simulink model "CTDSM_CIFF_SECOND_2048_RESIDUAL_OFFSET_CHOPPING"  (R2025b)
settings: Solver=VariableStepAuto  StartTime=0.0  StopTime=0.5  RelTol=1e-3
libraries: fl_lib x13, nesl_utility x6, ee_lib x2, simulink_extras x1, cstblocks x1, dspobslib x1
settings Model: Creator=Team_33  LastModifiedBy=k2vas

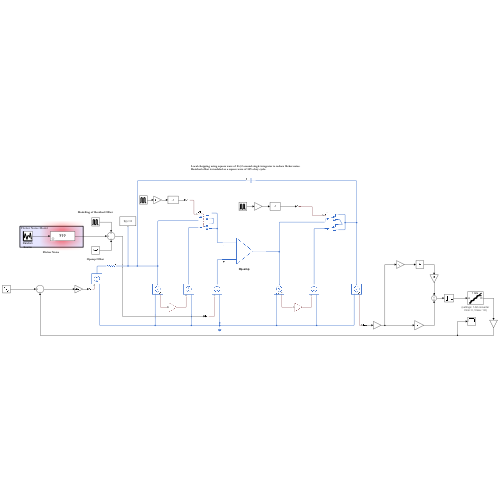
[thumbnail: Simulink's stored preview of the top-level diagram]
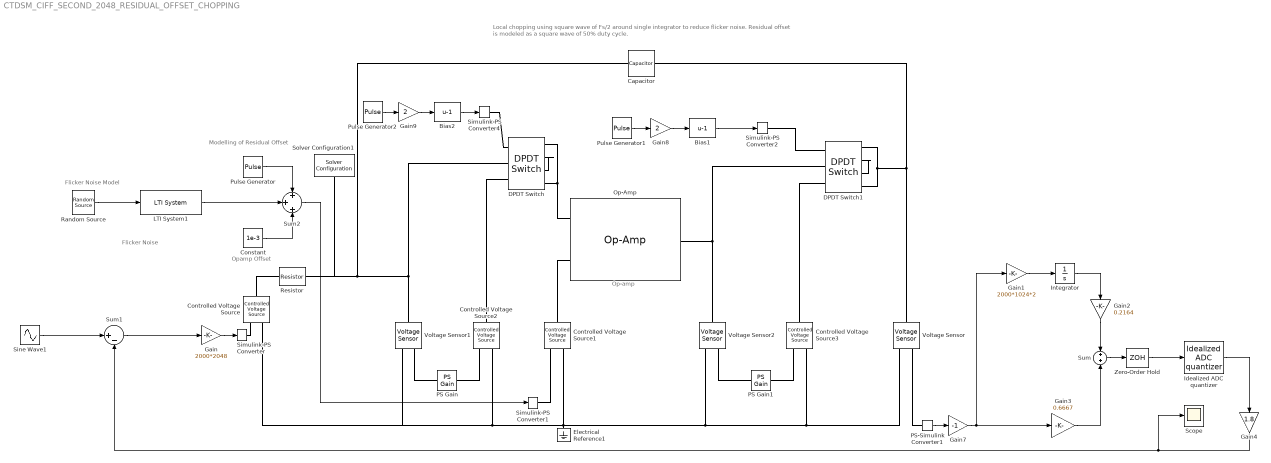
== system CTDSM_CIFF_SECOND_2048_RESIDUAL_OFFSET_CHOPPING ==
  note: Op-amp
  note: Local chopping using square wave of Fs/2 around single integrator to reduce flicker noise. Residual offset is modeled as a square wave of 50% duty cycle.
  note: Flicker Noise Model
  note: Opamp Offset
  note: Flicker Noise
  note: Modelling of Residual Offset
  Bias1 : Bias  Bias=-1  SaturateOnIntegerOverflow=off
  Bias2 : Bias  Bias=-1  SaturateOnIntegerOverflow=off
  Capacitor : fl_lib/Electrical/Electrical Elements/Capacitor  c=1 F  r=0 Ohm  g=0 1/Ohm  i_specify=off  i_priority=None  i=0 A  i_nominal_specify=off  i_nominal_value=1  i_nominal_unit=A  v_specify=off  v_priority=None  v=0 V  v_nominal_specify=off  v_nominal_value=1  v_nominal_unit=V  vc_specify=off  vc_priority=High  vc=0 V  vc_nominal_specify=off  vc_nominal_value=1  vc_nominal_unit=V
  Constant : Constant  Value=1e-3
  Controlled Voltage Source{,1..3} (4 alike) : fl_lib/Electrical/Electrical Sources/Controlled Voltage Source
  DPDT Switch : ee_lib/Switches & Breakers/DPDT Switch  R_closed=0.01 Ohm  G_open=1e-6 S  Threshold=0.5 V  Width=0 V  model_dynamics=0  t_on=1e-3 s  t_off=1e-3 s  initial_vT=0 V
      settings: InternalSimscapePortConfiguration="{\"Bottom\":[],\"Left\":[{\"id\":\"vT\",\"label\":\"vT\",\"type\":\"input\"},{\"id\":\"p1\",\"label\":\"\",\"type\":\"foundation.electrical.electrical\"},{\"id\":\"p2\",\"label\":\"\",\"type\":\"foundation.electrical.electrical\"}],\"Right\":[{\"id\":\"n11\",\"label\":\"\",\"type\":\"foundation.electrical.electrical\"},{\"id\":\"n12\",\"label\":\"\",\"type\":\"foundation.electrical.electrical\"},{\"id\":\"n21\",\"label\":\"\",\"type\":\"foundation.electrical.electrical\"},{\"id\":\"n22\",\"label\":\"\",\"type\":\"foundation.electrical.electrical\"}],\"Top\":[]}"
  DPDT Switch1 : ee_lib/Switches & Breakers/DPDT Switch  R_closed=0.01 Ohm  G_open=1e-6 S  Threshold=0.5 V  Width=0 V  model_dynamics=0  t_on=1e-3 s  t_off=1e-3 s  initial_vT=0 V
      settings: InternalSimscapePortConfiguration="{\"Bottom\":[],\"Left\":[{\"id\":\"vT\",\"label\":\"vT\",\"type\":\"input\"},{\"id\":\"p1\",\"label\":\"\",\"type\":\"foundation.electrical.electrical\"},{\"id\":\"p2\",\"label\":\"\",\"type\":\"foundation.electrical.electrical\"}],\"Right\":[{\"id\":\"n11\",\"label\":\"\",\"type\":\"foundation.electrical.electrical\"},{\"id\":\"n12\",\"label\":\"\",\"type\":\"foundation.electrical.electrical\"},{\"id\":\"n21\",\"label\":\"\",\"type\":\"foundation.electrical.electrical\"},{\"id\":\"n22\",\"label\":\"\",\"type\":\"foundation.electrical.electrical\"}],\"Top\":[]}"
  Electrical Reference1 : fl_lib/Electrical/Electrical Elements/Electrical Reference
  Gain : Gain  Gain=2000*2048
  Gain1 : Gain  Gain=2000*1024*2
  Gain2 : Gain  Gain=0.2164
  Gain3 : Gain  Gain=0.6667
  Gain4 : Gain  Gain=1.8
  Gain7 : Gain  Gain=-1
  Gain8 : Gain  Gain=2
  Gain9 : Gain  Gain=2
  Idealized ADC quantizer : simulink_extras/Additional Discrete/Idealized ADC quantizer  NumberOfConverterBits=1  Vmin=0  Vmax=1.8  OutputDataType=int16  OutputNegativeValues=off
  Integrator : Integrator
  LTI System1 : cstblocks/LTI System  sys=ff_ss  IC=[]  PadeOrder=0
  Op-Amp : fl_lib/Electrical/Electrical Elements/Op-Amp  outI_specify=off  outI_priority=None  outI=0 A  outI_nominal_specify=off  outI_nominal_value=1  outI_nominal_unit=A
  PS Gain : fl_lib/Physical Signals/Functions/PS Gain  gain=-1
  PS Gain1 : fl_lib/Physical Signals/Functions/PS Gain  gain=-1
  PS-Simulink Converter1 : nesl_utility/PS-Simulink Converter  PhysicalDomain=network_engine_domain  SubClassName=ps_output  LeftPortType=input  RightPortType=output  PseudoPeriodic=off  Frequencies=[]  VectorFormat=inherit  Unit=inherit  AffineConversion=off
  Pulse Generator : DiscretePulseGenerator  PulseType=Time based  Amplitude=2  Period=2/(2000*2048)  PulseWidth=50
  Pulse Generator1 : DiscretePulseGenerator  PulseType=Time based  Period=2/(2000*2048)  PulseWidth=50
  Pulse Generator2 : DiscretePulseGenerator  PulseType=Time based  Period=2/(2048*2000)  PulseWidth=50
  Random Source : dspobslib/Random Source  SrcType=Gaussian  NormMethod=Ziggurat  CltLength=12  MinVal=0  MaxVal=1  MeanVal=0  VarVal=1e-8  RepMode=Not repeatable  rawSeed=1  IsInherit=off  SampMode=Continuous  SampTime=1/(2000*2048)  SampFrame=1  DataType=Double  OutComplex=Real  OutputFrames=off
  Resistor : fl_lib/Electrical/Electrical Elements/Resistor  R=1 Ohm  i_specify=off  i_priority=None  i=0 A  i_nominal_specify=off  i_nominal_value=1  i_nominal_unit=A  v_specify=off  v_priority=None  v=0 V  v_nominal_specify=off  v_nominal_value=1  v_nominal_unit=V
  Scope : Scope
      settings: ActiveDisplayYMinimum=-0.225  ActiveDisplayYMaximum=2.02499  DataLoggingVariableName=output_data  DataLoggingSaveFormat=Array
  Simulink-PS Converter{,1..2,4} (4 alike) : nesl_utility/Simulink-PS Converter  PhysicalDomain=network_engine_domain  SubClassName=ps_input  LeftPortType=input  RightPortType=output  PseudoPeriodic=off  Frequencies=[]  NoiseDistribution=none  NoiseParameters=[]  Unit=1  AffineConversion=off  FilteringAndDerivatives=provide  SimscapeFilterOrder=1  InputFilterTimeConstant=0.001  UdotUserProvided=0
  Sine Wave1 : Sin  Amplitude=0.5  Bias=0.9  Frequency=((2000*1024)*127*2*2*pi)/(32768*32)  SampleTime=0
  Solver Configuration1 : nesl_utility/Solver Configuration  PhysicalDomain=network_engine_domain  SubClassName=solver  LeftPortType=input  RightPortType=generic  Tones=[]  Harmonics=[]  SimulateNoise=off  Profile=off  UseLocalSampling=off  EnableSwitchedLinearOptims=on  FrequencyDomain=off  UseCCode=off  RelTol=0.001  AbsTol=0.001  MinStep=1e-09  ToWorkspace=off  RevertToSquareIcSolve=off  NumHomotopyIterations=100  PhasorMode=off  PhasorModeNumHarmonics=1  ConsistencySolver=NEWTON_XTOL_AFTER_FTOL  IndexReductionMethod=DerivativeReplacement  DoDC=off  ResidualTolerance=1e-09  ConsistencyTolSource=GLOBAL  ConsistencyAbsTol=0.001  ConsistencyRelTol=0.001  ConsistencyTolFactor=0.001  UseLocalSolver=off  LocalSolverChoice=NE_BACKWARD_EULER_ADVANCER  ResolveIndetEquations=on  FunctionEvalNumThread=1  LocalSolverSampleTime=0.001  DoFixedCost=off  MaxNonlinIter=3  MaxModeIter=2  ComputeImpulses=off  ImpulseIterations=2  LinearAlgebra=auto  LinearAlgebraNumThread=0  EquationFormulation=NE_TIME_EF  DelaysMemoryBudget=1024  AutomaticFiltering=on  FilteringTimeConstant=0.001  PartitionStorageMethod=AS_NEEDED  PartitionMemoryBudget=1024  PartitionMethod=ROBUST  MultibodyUseLocalSolver=off  MultibodyLocalSolverChoice=ODE1  MultibodyLocalSolverSampleTime=0.001
  Sum : Sum  Inputs=+|+
  Sum1 : Sum  Inputs=|+-
  Sum2 : Sum  Inputs=+|+|+
  Voltage Sensor : fl_lib/Electrical/Electrical Sensors/Voltage Sensor
  Voltage Sensor1 : fl_lib/Electrical/Electrical Sensors/Voltage Sensor
  Voltage Sensor2 : fl_lib/Electrical/Electrical Sensors/Voltage Sensor
  Zero-Order Hold : ZeroOrderHold  SampleTime=1/(2000*1024*2)
  wires:
  Sum1/1 -> Gain/1
  Gain2/1 -> Sum/1
  Gain3/1 -> Sum/2
  Gain/1 -> Simulink-PS Converter/1
  PS-Simulink Converter1/1 -> Gain7/1
  Zero-Order Hold/1 -> Idealized ADC quantizer/1
  Idealized ADC quantizer/1 -> Gain4/1
  Gain1/1 -> Integrator/1
  Gain4/1 -> Scope/1, Sum1/2
  Integrator/1 -> Gain2/1
  Sum/1 -> Zero-Order Hold/1
  Sine Wave1/1 -> Sum1/1
  Gain7/1 -> Gain1/1, Gain3/1
  Bias1/1 -> Simulink-PS Converter2/1
  Pulse Generator1/1 -> Gain8/1
  Gain8/1 -> Bias1/1
  Pulse Generator2/1 -> Gain9/1
  Bias2/1 -> Simulink-PS Converter4/1
  Gain9/1 -> Bias2/1
  Random Source/1 -> LTI System1/1
  LTI System1/1 -> Sum2/2
  Pulse Generator/1 -> Sum2/1
  Sum2/1 -> Simulink-PS Converter1/1
  Constant/1 -> Sum2/3
  connections:
  DPDT Switch1/RConn1 -- DPDT Switch1/RConn4 -- Capacitor/RConn1 -- Voltage Sensor/LConn1
  Controlled Voltage Source/LConn1 -- Resistor/LConn1
  PS-Simulink Converter1/LConn1 -- Voltage Sensor/RConn1
  Controlled Voltage Source/RConn1 -- Simulink-PS Converter/RConn1
  Voltage Sensor/RConn2 -- Controlled Voltage Source3/RConn2 -- Voltage Sensor2/RConn2 -- Electrical Reference1/LConn1 -- Controlled Voltage Source1/RConn2 -- Voltage Sensor1/RConn2 -- Controlled Voltage Source/RConn2 -- Controlled Voltage Source2/RConn2
  DPDT Switch/RConn1 -- Op-Amp/LConn2 -- DPDT Switch/RConn4
  DPDT Switch/RConn2 -- DPDT Switch/RConn3
  Simulink-PS Converter4/RConn1 -- DPDT Switch/LConn1
  DPDT Switch1/LConn1 -- Simulink-PS Converter2/RConn1
  Voltage Sensor1/RConn1 -- PS Gain/LConn1
  PS Gain/RConn1 -- Controlled Voltage Source2/RConn1
  Voltage Sensor2/RConn1 -- PS Gain1/LConn1
  PS Gain1/RConn1 -- Controlled Voltage Source3/RConn1
  DPDT Switch1/RConn2 -- DPDT Switch1/RConn3
  Controlled Voltage Source1/LConn1 -- Op-Amp/LConn1
  Controlled Voltage Source1/RConn1 -- Simulink-PS Converter1/RConn1
  Voltage Sensor1/LConn1 -- DPDT Switch/LConn2 -- Capacitor/LConn1 -- Solver Configuration1/RConn1 -- Resistor/RConn1
  Controlled Voltage Source2/LConn1 -- DPDT Switch/LConn3
  Controlled Voltage Source3/LConn1 -- DPDT Switch1/LConn3
  Voltage Sensor2/LConn1 -- Op-Amp/RConn1 -- DPDT Switch1/LConn2
